simulink library "tqr"  (R2021b)
settings: Solver=VariableStepAuto  StartTime=0.0  StopTime=10.0  RelTol=1e-3
undefined symbols (not defined in the file): ATQR_AltRDCActiveFEDUInc_X_pct, ATQR_AltRDCActiveFEDUInc_Y_enum, ATQR_AltRDCActiveFEDUTs_X_pct, ATQR_AltRDCActiveFEDUTs_Y_enum, ATQR_AltRDCActiveREDUInc_X_pct, ATQR_AltRDCActiveREDUInc_Y_enum, ATQR_AltRDCActiveREDUTs_X_pct, ATQR_AltRDCActiveREDUTs_Y_enum, ATQR_CreepFEDUTqIncSR_X_rpm, ATQR_CreepFEDUTqIncSR_Y_Nm, ATQR_CreepFEDUTs_X_rpm, ATQR_CreepFEDUTs_Y_Nm, ATQR_ECO2TqFrIncGain_X_Nm, ATQR_ECO2TqFrIncGain_Y_pct, ATQR_ECO2TqRrIncGain_X_Nm, ATQR_ECO2TqRrIncGain_Y_pct, ATQR_EcoTqFrIncGain_X_Nm, ATQR_EcoTqFrIncGain_Y_pct, ATQR_EcoTqRrIncGain_X_Nm, ATQR_EcoTqRrIncGain_Y_pct, ATQR_EL1FEDUTqDecSR_Y_Nm, ATQR_EL1FEDUTqIncSR_X_rpm, ATQR_EL1FEDUTqIncSR_Y_pct, ATQR_EL1FEDUTs_X_rpm, ATQR_EL1FEDUTs_Y_Nm, ATQR_EL1REDUTqDecSR_Y_Nm, ATQR_EL1REDUTs_Y_Nm, ATQR_FEDUEL1RegenTs_X_rpm, ATQR_FEDUTIPOutTs_X_rpm, ATQR_FrNegRateLimitIncN_X_rpm, ATQR_FrNegRateLimitIncN_Y_Nm, ATQR_FrPosRateLimitIncN_X_rpm, ATQR_FrPosRateLimitIncN_Y_Nm, ATQR_FrPreLoadTqIncSR_X_rpm, ATQR_FrPreLoadTqIncSR_Y_Nm, ATQR_FShaftSpdTqLimCoe_X_rpm, ATQR_FTimerTqLimCoe_X_s, ATQR_FTqZeroTransUpBoundN_X_rpm, ATQR_NL1FEDUTqDecSR_Y_Nm, ATQR_NL1FEDUTqIncSR_X_rpm, ATQR_NL1FEDUTqIncSR_Y_pct, ATQR_NL1FEDUTs_X_rpm, ATQR_NL1FEDUTs_Y_Nm, ATQR_NL1REDUTqDecSR_Y_Nm, ATQR_NL1REDUTs_Y_Nm, ATQR_NL2TqFrIncGain_X_Nm, ATQR_NL2TqFrIncGain_Y_pct, ATQR_NL2TqRrIncGain_X_Nm, ATQR_NL2TqRrIncGain_Y_pct, ATQR_NormalTqFrIncGain_X_Nm, ATQR_NormalTqFrIncGain_Y_pct, ATQR_NormalTqRrIncGain_X_Nm, ATQR_NormalTqRrIncGain_Y_pct, ATQR_RrNegRateLimitIncN_X_rpm, ATQR_RrNegRateLimitIncN_Y_Nm, ATQR_RrPosRateLimitIncN_X_rpm, ATQR_RrPosRateLimitIncN_Y_Nm, ATQR_RrPreLoadTqIncSR_X_rpm, ATQR_RrPreLoadTqIncSR_Y_Nm, ATQR_RShaftSpdTqLimCoe_X_rpm ... (+349)
libraries: hcu_lib x21, simulink x15, $bdroot x3
(part 2 of 12)

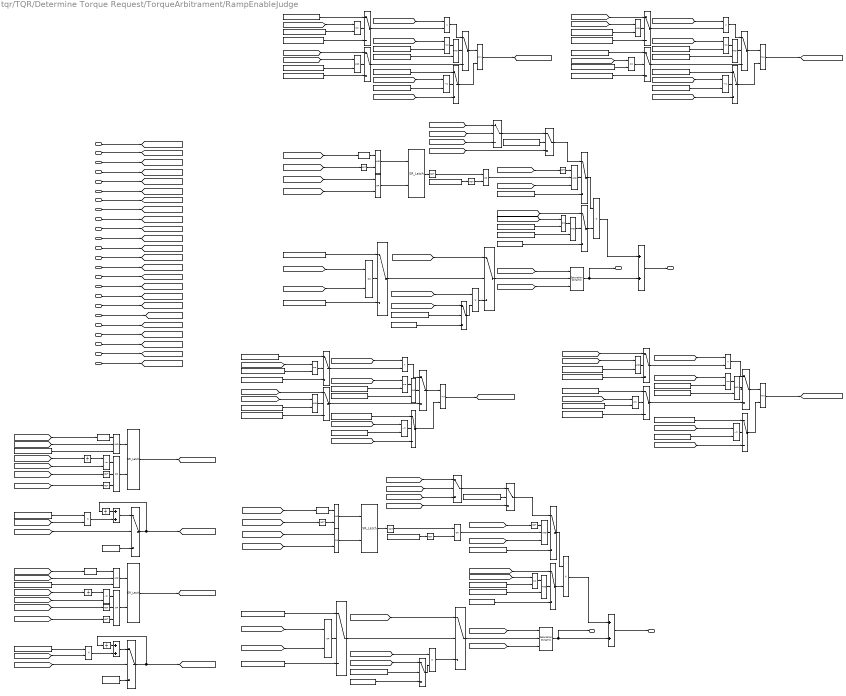
== system tqr/TQR/Determine Torque Request/TorqueArbitrament/RampEnableJudge ==
  VTQD_AfterAvailableTqDemFr_Nm : Inport
  VINP_FrPTCSActive_flg : Inport  Port=2
  VINP_FrRBCActive_flg : Inport  Port=3
  VINP_ADASForceIdle_flg : Inport  Port=4
  VTQR_RampFEDUWhlTqReq_Nm : Inport  Port=5
  VTQD_AfterAvailableTqDemRr_Nm : Inport  Port=6
  VINP_RrPTCSActive_flg : Inport  Port=7
  VINP_RrRBCActive_flg : Inport  Port=8
  VTQR_RampREDUWhlTqReq_Nm : Inport  Port=9
  VTQD_LoSpdBrkCtrl_flg : Inport  Port=10
  VTQD_RDCActive_enum : Inport  Port=11
  VINP_FrntAxlTrqReqBrk_Nm : Inport  Port=12
  VINP_RearAxlTrqReqBrk_Nm : Inport  Port=13
  VVMC_ADASActive_flg : Inport  Port=14
  VINP_FrntAxlTrqReqDrv_Nm : Inport  Port=15
  VINP_RearAxlTrqReqDrv_Nm : Inport  Port=16
  VTQR_RampTqCMDGain_c : Inport  Port=17
  VTQD_GearActualPosn_enum : Inport  Port=18
  VTQD_BrkSwSta_flg : Inport  Port=19
  task_time_s : Inport  Port=20
  VTQD_WhlTqCapMotFr_Nm : Inport  Port=21
  VTQD_WhlTqCapMotRr_Nm : Inport  Port=22
  VTQD_WhlTqCapGenFr_Nm : Inport  Port=23
  VTQD_WhlTqCapGenRr_Nm : Inport  Port=24
  AND{,1..2,4,6..7,10,12,18..21} (12 alike) : Logic  AllPortsSameDT=off  OutDataTypeStr=boolean
  AND{8..9,11,13} (4 alike) : Logic  Operator=OR  AllPortsSameDT=off  OutDataTypeStr=boolean
  AND{3,5,14,16} (4 alike) : Logic  Inputs=3  AllPortsSameDT=off  OutDataTypeStr=boolean
  AND15 : Logic  Operator=OR  Inputs=3  AllPortsSameDT=off  OutDataTypeStr=boolean
  AND17 : Logic  Operator=OR  Inputs=3  AllPortsSameDT=off  OutDataTypeStr=boolean
  Add{,1..3} (4 alike) : Sum
  Constant : Constant  Value=TRUE
  Constant1 : Constant  Value=FALSE
  Constant{10,12,14,22} (4 alike) : Constant  Value=ONE_INT
  Constant{6,11,18,28} (4 alike) : Constant  Value=ENUM_CANRDCACTSTA_EXITIMMEDIATELY
  Constant{9,13,15..16,20,24,26,30} (8 alike) : Constant  Value=KTQR_NewRampArchSW_flg
  Constant{17,21,23,25,27,31} (6 alike) : Constant  Value=ENUM_GEARACTUALPOSN_R
  Constant{4..5,7..8,19,29,34,39} (8 alike) : Constant  Value=ZERO_FLOAT
  Constant2 : Constant  Value=TRUE
  Constant3 : Constant  Value=FALSE
  Constant32 : Constant  Value=KTQR_ACCCancelNoRBC_flg
  Constant33 : Constant  Value=KTQR_ACCCancelNoRBC_flg
  Constant35 : Constant  Value=KTQR_ADASCancelBRgnSlopeF_Nmps
  Constant{36..38,41} (4 alike) : Constant  Value=KTQR_ADASCancelBRgnSlopeSW_flg
  Constant40 : Constant  Value=KTQR_ADASCancelBRgnSlopeR_Nmps
  Constant{42..44,46} (4 alike) : Constant  Value=ENUM_GEARACTUALPOSN_D
  Constant45 : Constant  Value=KTQR_FinalFEDUTrqLowLim_Nm
  Constant47 : Constant  Value=KTQR_FinalFEDUTrqUpLim_Nm
  Detect Decrease{,1..3} (4 alike) : simulink/Logic and Bit Operations/Detect Decrease  vinit=0.0  OutDataTypeStr=boolean
  Divide : Product  Inputs=**
  Divide1 : Product  Inputs=**
  Equal{,1..9} (10 alike) : RelationalOperator  Operator===  OutDataTypeStr=boolean  RndMeth=Simplest
  Equal{10..13} (4 alike) : RelationalOperator  Operator=~=  OutDataTypeStr=boolean  RndMeth=Simplest
  Logical Operator1 : Logic  Operator=OR  AllPortsSameDT=off  OutDataTypeStr=boolean
  Logical Operator2 : Logic  Operator=OR  AllPortsSameDT=off  OutDataTypeStr=boolean
  Min : MinMax  Inputs=2
  Min1 : MinMax  Function=max  Inputs=2
  Min2 : MinMax  Inputs=2
  Min3 : MinMax  Function=max  Inputs=2
  NOT{,1..11} (12 alike) : Logic  Operator=NOT  AllPortsSameDT=off  OutDataTypeStr=boolean
  Product{,1..7} (8 alike) : Product
  RegenLV_inc1 : Constant  Value=KTQR_FinalFEDUTrqLowLim_Nm  OutDataTypeStr=single
  RegenLV_inc{9..12} (4 alike) : Constant  Value=KTQR_TCSActTQRLimSW_flg  OutDataTypeStr=single
  RegenLV_inc13 : Constant  Value=KTQR_FinalREDUTrqUpLim_Nm  OutDataTypeStr=single
  RegenLV_inc14 : Constant  Value=KTQR_FinalREDUTrqLowLim_Nm  OutDataTypeStr=single
  RegenLV_inc2 : Constant  Value=KTQR_FinalFEDUTrqUpLim_Nm  OutDataTypeStr=single
  RegenLV_inc3 : Constant  Value=KTQR_FinalREDUTrqLowLim_Nm  OutDataTypeStr=single
  RegenLV_inc4 : Constant  Value=KTQR_FinalREDUTrqUpLim_Nm  OutDataTypeStr=single
  RegenLV_inc5 : Constant  Value=KTQR_FinalFEDUTrqUpLim_Nm  OutDataTypeStr=single
  RegenLV_inc6 : Constant  Value=KTQR_FinalFEDUTrqLowLim_Nm  OutDataTypeStr=single
  RegenLV_inc7 : Constant  Value=KTQR_FinalREDUTrqUpLim_Nm  OutDataTypeStr=single
  RegenLV_inc8 : Constant  Value=KTQR_FinalREDUTrqLowLim_Nm  OutDataTypeStr=single
  Relational Operator : RelationalOperator  Operator=<=  OutDataTypeStr=boolean  RndMeth=Simplest
  Relational Operator1 : RelationalOperator  Operator=<=  OutDataTypeStr=boolean  RndMeth=Simplest
  SR_Latch{1..4} (4 alike) : hcu_lib/Basic_Blocks/SR_Latch
  Saturation Dynamic : simulink/Discontinuities/Saturation Dynamic  OutMin=[]  OutMax=[]  OutDataTypeStr=Inherit: Same as second input  OutDataType=fixdt(1, 16)  OutScaling=2^-10  DoSatur=off
  Saturation Dynamic1 : simulink/Discontinuities/Saturation Dynamic  OutMin=[]  OutMax=[]  OutDataTypeStr=Inherit: Same as second input  OutDataType=fixdt(1, 16)  OutScaling=2^-10  DoSatur=off
  Switch{,1..5} (6 alike) : Switch  Criteria=u2 ~= 0
  Switch{6..31} (26 alike) : Switch  Criteria=u2 > Threshold
  Unit Delay{,1..3} (4 alike) : UnitDelay  SampleTime=-1  HasFrameUpgradeWarning=on
  VTQR_ActualFEDUWhlTqReq_Nm : Outport
  VTQR_ActualREDUWhlTqReq_Nm : Outport  Port=2
  VTQR_NoABSFEDUWhlTqReq_Nm : Outport  Port=3
  VTQR_NoABSREDUWhlTqReq_Nm : Outport  Port=4
  wires:
  VINP_ADASForceIdle_flg/1 -> [VINP_ADASForceIdle_flg]
  VINP_FrPTCSActive_flg/1 -> [VINP_FrPTCSActive_flg]
  VINP_RrPTCSActive_flg/1 -> [VINP_RrPTCSActive_flg]
  VINP_FrRBCActive_flg/1 -> [VINP_FrRBCActive_flg]
  VINP_RrRBCActive_flg/1 -> [VINP_RrRBCActive_flg]
  VTQD_LoSpdBrkCtrl_flg/1 -> [VTQD_LoSpdBrkCtrl_flg]
  VTQD_RDCActive_enum/1 -> [VTQD_RDCActive_enum]
  VINP_FrntAxlTrqReqBrk_Nm/1 -> [VINP_FrntAxlTrqReqBrk_Nm]
  VINP_RearAxlTrqReqBrk_Nm/1 -> [VINP_RearAxlTrqReqBrk_Nm]
  VTQR_RampFEDUWhlTqReq_Nm/1 -> [VTQR_RampFEDUWhlTqReq_Nm]
  VTQR_RampREDUWhlTqReq_Nm/1 -> [VTQR_RampREDUWhlTqReq_Nm]
  VVMC_ADASActive_flg/1 -> [VVMC_ADASActive_flg]
  VTQD_AfterAvailableTqDemFr_Nm/1 -> [VTQD_AfterAvailableTqDemFr_Nm]
  VTQD_AfterAvailableTqDemRr_Nm/1 -> [VTQD_AfterAvailableTqDemRr_Nm]
  VINP_RearAxlTrqReqDrv_Nm/1 -> [VINP_RearAxlTrqReqDrv_Nm]
  VINP_FrntAxlTrqReqDrv_Nm/1 -> [VINP_FrntAxlTrqReqDrv_Nm]
  Constant7/1 -> Switch6/1
  [VINP_ADASForceIdle_flg] -> Logical Operator1/1
  Constant2/1 -> Switch3/3
  Constant6/1 -> Equal/2
  RegenLV_inc2/1 -> Switch8/3
  Constant1/1 -> Switch2/1
  [VTQR_RampREDUWhlTqReq_Nm] -> Switch1/1
  Switch2/1 -> Switch/2  "VTQR_FrRampEnable_flg"
  Constant3/1 -> Switch3/1
  Logical Operator1/1 -> Switch2/2
  RegenLV_inc4/1 -> Switch9/3
  Constant8/1 -> Switch7/1
  Equal4/1 -> Switch7/2
  Constant11/1 -> Equal4/2
  [VTQD_RDCActive_enum] -> Equal/1
  [VINP_FrntAxlTrqReqDrv_Nm] -> Switch8/1
  Constant5/1 -> Switch5/3
  Equal/1 -> Switch6/2
  Switch3/1 -> Switch1/2  "VTQR_RrRampEnable_flg"
  [VTQD_RDCActive_enum] -> Equal4/1
  NOT1/1 -> AND3/1
  Logical Operator2/1 -> Switch3/2
  [VINP_RearAxlTrqReqDrv_Nm] -> Switch9/1
  [VTQR_RampFEDUWhlTqReq_Nm] -> Switch/1
  Constant/1 -> Switch2/3
  [VVMC_ADASActive_flg] -> NOT2/1
  NOT2/1 -> AND5/1
  AND3/1 -> Switch4/2
  AND5/1 -> Switch5/2
  [VVMC_ADASActive_flg] -> NOT1/1
  [VINP_RrRBCActive_flg] -> AND5/3
  Constant4/1 -> Switch4/3
  Switch1/1 -> Saturation Dynamic1/2
  RegenLV_inc1/1 -> Switch6/3
  [VINP_FrRBCActive_flg] -> AND3/3
  RegenLV_inc3/1 -> Switch7/3
  [VINP_ADASForceIdle_flg] -> Logical Operator2/1
  [VTQD_LoSpdBrkCtrl_flg] -> Logical Operator1/2
  [VTQD_LoSpdBrkCtrl_flg] -> Logical Operator2/2
  VTQR_RampTqCMDGain_c/1 -> [VTQR_RampTqCMDGain_c]
  Product/1 -> Switch/3
  [VTQD_AfterAvailableTqDemFr_Nm] -> Product/1
  Switch10/1 -> Product/2
  [VTQR_RampTqCMDGain_c] -> Switch10/1
  Constant9/1 -> Switch10/2
  Constant10/1 -> Switch10/3
  Constant13/1 -> Switch11/2
  Switch11/1 -> Product1/2
  Constant12/1 -> Switch11/3
  Product1/1 -> Switch1/3
  [VTQD_AfterAvailableTqDemRr_Nm] -> Product1/1
  [VTQR_RampTqCMDGain_c] -> Switch11/1
  Constant14/1 -> Switch12/3
  [VTQR_RampTqCMDGain_c] -> Switch12/1
  Switch12/1 -> Product2/2
  Product2/1 -> Add/1
  Switch4/1 -> Product2/1
  [VTQR_ActFEDUTqLowLimit_Nm] -> Saturation Dynamic/3
  Switch6/1 -> Switch13/3
  AND/1 -> Switch13/2
  Constant16/1 -> AND/2
  VTQD_GearActualPosn_enum/1 -> [VTQD_GearActualPosn_enum]
  Equal1/1 -> AND/1
  [VTQD_GearActualPosn_enum] -> Equal1/1
  Constant17/1 -> Equal1/2
  [VINP_FrntAxlTrqReqDrv_Nm] -> Switch14/1
  RegenLV_inc5/1 -> Switch14/3
  Product3/1 -> Switch13/1
  Switch14/1 -> Product3/2
  [VTQR_RampTqCMDGain_c] -> Product3/1
  Equal2/1 -> Switch15/2
  RegenLV_inc6/1 -> Switch15/3
  [VTQD_RDCActive_enum] -> Equal2/1
  Constant18/1 -> Equal2/2
  Constant19/1 -> Switch15/1
  [VTQR_RampTqCMDGain_c] -> Product4/1
  AND1/1 -> Switch16/2
  Equal3/1 -> AND1/1
  Constant21/1 -> Equal3/2
  Product4/1 -> Switch16/1
  Constant20/1 -> AND1/2
  [VTQD_GearActualPosn_enum] -> Equal3/1
  Switch15/1 -> Product4/2
  Switch8/1 -> Switch16/3
  [VTQR_RampTqCMDGain_c] -> Switch17/1
  Constant22/1 -> Switch17/3
  Switch5/1 -> Product5/1
  Product5/1 -> Add1/1
  [VTQR_ActREDUTqLowLimit_Nm] -> Saturation Dynamic1/3
  [VTQR_RampTqCMDGain_c] -> Product6/1
  AND2/1 -> Switch18/2
  Equal5/1 -> AND2/1
  Constant25/1 -> Equal5/2
  Product6/1 -> Switch18/1
  Constant24/1 -> AND2/2
  [VTQD_GearActualPosn_enum] -> Equal5/1
  Switch19/1 -> Product6/2
  Switch7/1 -> Switch18/3
  [VINP_RearAxlTrqReqDrv_Nm] -> Switch19/1
  RegenLV_inc7/1 -> Switch19/3
  Product7/1 -> Switch20/1
  Constant27/1 -> Equal6/2
  [VTQD_GearActualPosn_enum] -> Equal6/1
  Equal6/1 -> AND4/1
  Constant26/1 -> AND4/2
  [VTQR_RampTqCMDGain_c] -> Product7/1
  Switch21/1 -> Product7/2
  AND4/1 -> Switch20/2
  Switch9/1 -> Switch20/3
  [VTQR_ActREDUTqUpLimit_Nm] -> Saturation Dynamic1/1
  [VTQR_ActFEDUTqUpLimit_Nm] -> Saturation Dynamic/1
  RegenLV_inc8/1 -> Switch21/3
  Constant29/1 -> Switch21/1
  Equal7/1 -> Switch21/2
  Constant28/1 -> Equal7/2
  [VTQD_RDCActive_enum] -> Equal7/1
  Switch17/1 -> Product5/2
  Equal8/1 -> AND6/1
  Constant23/1 -> Equal8/2
  Constant15/1 -> AND6/2
  [VTQD_GearActualPosn_enum] -> Equal8/1
  AND6/1 -> Switch17/2
  Constant30/1 -> AND7/2
  [VTQD_GearActualPosn_enum] -> Equal9/1
  Constant31/1 -> Equal9/2
  Equal9/1 -> AND7/1
  AND7/1 -> Switch12/2
  NOT3/1 -> AND8/2
  Constant32/1 -> NOT3/1
  AND8/1 -> AND3/2
  Constant33/1 -> NOT4/1
  NOT4/1 -> AND9/2
  AND9/1 -> AND5/2
  VTQD_BrkSwSta_flg/1 -> [VTQD_BrkSwSta_flg]
  [VVMC_ADASActive_flg] -> Detect Decrease/1
  [VTQD_BrkSwSta_flg] -> NOT/1
  AND10/1 -> SR_Latch1/1
  Detect Decrease/1 -> AND10/1
  [VVMC_ADASActive_flg] -> AND11/1
  NOT/1 -> AND10/2
  [VTQD_BrkSwSta_flg] -> AND11/2
  AND11/1 -> SR_Latch1/2
  SR_Latch1/1 -> NOT6/1
  [VTQD_BrkSwSta_flg] -> AND13/2
  [VTQD_BrkSwSta_flg] -> NOT5/1
  AND13/1 -> SR_Latch2/2
  NOT5/1 -> AND12/2
  Detect Decrease1/1 -> AND12/1
  [VVMC_ADASActive_flg] -> Detect Decrease1/1
  AND12/1 -> SR_Latch2/1
  [VVMC_ADASActive_flg] -> AND13/1
  SR_Latch2/1 -> NOT7/1
  NOT6/1 -> AND9/1
  NOT7/1 -> AND8/1
  Switch26/1 -> Switch23/1
  [VINP_FrntAxlTrqReqBrk_Nm] -> Switch26/3
  Constant37/1 -> Switch23/2
  [VTQR_FrntAxlTrqReqBrkRamp_Nm] -> Switch26/1
  [VTQR_ADASCancelBRgnRampF_flg] -> Switch26/2
  [VINP_FrntAxlTrqReqBrk_Nm] -> Switch23/3
  Relational Operator/1 -> AND15/1
  Unit Delay1/1 -> Add3/1
  Constant41/1 -> AND16/3
  Add2/1 -> Switch22/1
  SR_Latch4/1 -> [VTQR_ADASCancelBRgnRampR_flg]  "VTQR_ADASCancelBRgnRampR_flg"
  Constant40/1 -> Divide1/1
  AND16/1 -> SR_Latch4/1
  Constant35/1 -> Divide/1
  SR_Latch3/1 -> [VTQR_ADASCancelBRgnRampF_flg]  "VTQR_ADASCancelBRgnRampF_flg"
  [task_time_s] -> Divide1/2
  [VTQR_RearAxlTrqReqBrkRamp_Nm] -> Unit Delay3/1
  [VINP_RearAxlTrqReqBrk_Nm] -> Relational Operator1/2
  NOT10/1 -> AND17/2
  Switch22/1 -> Unit Delay/1, [VTQR_FrntAxlTrqReqBrkRamp_Nm]  "VTQR_FrntAxlTrqReqBrkRamp_Nm"
  NOT11/1 -> AND17/3
  AND17/1 -> SR_Latch4/2
  AND15/1 -> SR_Latch3/2
  NOT8/1 -> AND15/2
  Unit Delay/1 -> Add2/1
  [VTQR_FrntAxlTrqReqBrkRamp_Nm] -> Unit Delay2/1
  Divide/1 -> Add2/2
  Constant36/1 -> AND14/3
  Constant34/1 -> Switch22/3
  AND14/1 -> SR_Latch3/1
  Detect Decrease2/1 -> AND14/1
  [VTQR_ADASCancelBRgnRampF_flg] -> Switch22/2
  Unit Delay3/1 -> Relational Operator1/1
  Switch25/1 -> Unit Delay1/1, [VTQR_RearAxlTrqReqBrkRamp_Nm]  "VTQR_RearAxlTrqReqBrkRamp_Nm"
  Unit Delay2/1 -> Relational Operator/1
  [VTQR_ADASCancelBRgnRampR_flg] -> Switch25/2
  Constant39/1 -> Switch25/3
  NOT9/1 -> AND15/3
  [VVMC_ADASActive_flg] -> Detect Decrease3/1
  Add3/1 -> Switch25/1
  Relational Operator1/1 -> AND17/1
  [VINP_RrRBCActive_flg] -> NOT11/1
  Divide1/1 -> Add3/2
  Detect Decrease3/1 -> AND16/1
  [task_time_s] -> Divide/2
  [VVMC_ADASActive_flg] -> Detect Decrease2/1
  [VTQD_BrkSwSta_flg] -> AND14/2
  [VINP_FrntAxlTrqReqBrk_Nm] -> Relational Operator/2
  [VTQD_BrkSwSta_flg] -> NOT8/1
  [VINP_FrRBCActive_flg] -> NOT9/1
  [VTQD_BrkSwSta_flg] -> AND16/2
  [VTQD_BrkSwSta_flg] -> NOT10/1
  Constant38/1 -> Switch24/2
  [VINP_RearAxlTrqReqBrk_Nm] -> Switch27/3
  Switch27/1 -> Switch24/1
  [VTQR_RearAxlTrqReqBrkRamp_Nm] -> Switch27/1
  [VTQR_ADASCancelBRgnRampR_flg] -> Switch27/2
  [VINP_RearAxlTrqReqBrk_Nm] -> Switch24/3
  Add/1 -> VTQR_ActualFEDUWhlTqReq_Nm/1  "VTQR_ActualFEDUWhlTqReq_Nm"
  Switch/1 -> Saturation Dynamic/2
  Saturation Dynamic/1 -> Add/2, VTQR_NoABSFEDUWhlTqReq_Nm/1  "VTQR_NoABSFEDUWhlTqReq_Nm"
  Saturation Dynamic1/1 -> Add1/2, VTQR_NoABSREDUWhlTqReq_Nm/1  "VTQR_NoABSREDUWhlTqReq_Nm"
  Add1/1 -> VTQR_ActualREDUWhlTqReq_Nm/1  "VTQR_ActualREDUWhlTqReq_Nm"
  task_time_s/1 -> [task_time_s]
  Switch16/1 -> Min/1
  Min/1 -> [VTQR_ActFEDUTqUpLimit_Nm]  "VTQR_ActFEDUTqUpLimit_Nm"
  VTQD_WhlTqCapMotFr_Nm/1 -> [VTQD_WhlTqCapMotFr_Nm]
  VTQD_WhlTqCapMotRr_Nm/1 -> [VTQD_WhlTqCapMotRr_Nm]
  VTQD_WhlTqCapGenFr_Nm/1 -> [VTQD_WhlTqCapGenFr_Nm]
  VTQD_WhlTqCapGenRr_Nm/1 -> [VTQD_WhlTqCapGenRr_Nm]
  Switch13/1 -> Min1/1
  Min1/1 -> [VTQR_ActFEDUTqLowLimit_Nm]  "VTQR_ActFEDUTqLowLimit_Nm"
  Switch20/1 -> Min2/1
  Min2/1 -> [VTQR_ActREDUTqUpLimit_Nm]  "VTQR_ActREDUTqUpLimit_Nm"
  Switch18/1 -> Min3/1
  Min3/1 -> [VTQR_ActREDUTqLowLimit_Nm]  "VTQR_ActREDUTqLowLimit_Nm"
  AND18/1 -> Switch8/2
  [VINP_FrPTCSActive_flg] -> AND18/1
  RegenLV_inc9/1 -> AND18/2
  RegenLV_inc10/1 -> AND19/2
  AND19/1 -> Switch14/2
  [VINP_FrPTCSActive_flg] -> AND19/1
  RegenLV_inc11/1 -> AND20/2
  AND20/1 -> Switch19/2
  [VINP_RrPTCSActive_flg] -> AND20/1
  RegenLV_inc12/1 -> AND21/2
  AND21/1 -> Switch9/2
  [VINP_RrPTCSActive_flg] -> AND21/1
  [VTQD_WhlTqCapMotRr_Nm] -> Switch28/3
  Switch28/1 -> Min2/2
  Equal10/1 -> Switch28/2
  [VTQD_GearActualPosn_enum] -> Equal10/1
  Constant42/1 -> Equal10/2
  RegenLV_inc13/1 -> Switch28/1
  [VTQD_GearActualPosn_enum] -> Equal11/1
  Equal11/1 -> Switch29/2
  RegenLV_inc14/1 -> Switch29/1
  Constant43/1 -> Equal11/2
  [VTQD_WhlTqCapGenRr_Nm] -> Switch29/3
  Switch29/1 -> Min3/2
  [VTQD_GearActualPosn_enum] -> Equal12/1
  Equal12/1 -> Switch30/2
  Constant45/1 -> Switch30/1
  Constant44/1 -> Equal12/2
  [VTQD_WhlTqCapGenFr_Nm] -> Switch30/3
  Switch30/1 -> Min1/2
  Constant46/1 -> Equal13/2
  Equal13/1 -> Switch31/2
  [VTQD_GearActualPosn_enum] -> Equal13/1
  Constant47/1 -> Switch31/1
  [VTQD_WhlTqCapMotFr_Nm] -> Switch31/3
  Switch31/1 -> Min/2
  Switch24/1 -> Switch5/1
  Switch23/1 -> Switch4/1
